simulink model "problem2_2"  (R2020a)
settings: Solver=VariableStepAuto  StartTime=0.0  StopTime=10.0  MaxStep=0.0001  RelTol=1e-3
settings Model: Creator=dinhm  LastModifiedBy=dinhm

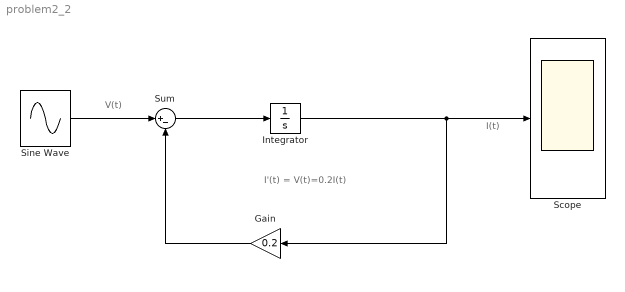
== system problem2_2 ==
  note: I(t)
  note: V(t)
  note: I'(t) = V(t)=0.2I(t)
  Gain : Gain  Gain=0.2
  Integrator : Integrator
  Scope : Scope
  Sine Wave : Sin  Amplitude=10  Phase=pi/4  SampleTime=0
  Sum : Sum  Inputs=|+-
  wires:
  Sine Wave/1 -> Sum/1
  Gain/1 -> Sum/2
  Sum/1 -> Integrator/1
  Integrator/1 -> Gain/1, Scope/1
